simulink library "microgridLib"  (R2023a)
settings: Solver=VariableStepAuto  StartTime=0.0  StopTime=10.0  RelTol=1e-3
values from neighbouring files (symbols this model uses):
  Ts = 5.0E-5    [microgrid_system.sldd]
  Ts_Control = 5.0E-5    [microgrid_system.sldd]
undefined symbols (not defined in the file or in its folder): BR, D1, Delta, DiscIntNeverNeededParam, fnom, gcbh, I1_init, Ion, j, Lithium, Mag_V0, np, nq, Pha_V0, PQext, sps_rtmsupport, Tp1, Tp2, Tq1, Tq2, Vbase, Vmin, Vnom
libraries: slpidlib x11, spsThreePhaseSeriesRLCBranchLib x10, spsGroundLib x9, spsVoltageMeasurementLib x7, spsSeriesRLCBranchLib x7, spsControlledCurrentSourceLib x6, spsabctodq0Lib x6, spsFourierLib x5, spsPower3phInstantaneousLib x5, spsThreePhaseSeriesRLCLoadLib x4, spsThreePhaseTransformerTwoWindingsLib x4, spsThreePhaseVIMeasurementLib x3
(part 2 of 4)

== system microgridLib/Transformer ==
  Ground : spsGroundLib/Ground  LConnTagsString=a
  Shunt (Numerical Stability) : spsThreePhaseSeriesRLCBranchLib/Three-Phase Series RLC Branch  LConnTagsString=A|B|C  RConnTagsString=A|B|C  BranchType=R  Resistance=1e7  Inductance=1e-3  Capacitance=1e-6  Measurements=None
  Three-Phase Transformer (Two Windings) : spsThreePhaseTransformerTwoWindingsLib/Three-Phase Transformer (Two Windings)  Winding1Connection=Delta (D1)  Winding2Connection=Yg  CoreType=Three single-phase transformers  SetSaturation=off  Hysteresis=off  DataFile='hysteresis'  SetInitialFlux=off  Measurements=None  UNITS=pu  NominalPower=[S Freq]  Winding1=[Vp 0 0]  Winding2=[Vs Z/Ratio Z/(2*pi*Freq)]  Rm=500  Lm=500  L0=0.5  Saturation=[ 0,0 ; 0.0024,1.2 ; 1.0,1.52 ]  InitialFluxes=[ 0.8 , -0.8 , 0.7 ]  BreakLoop=off  DiscreteSolver=Trapezoidal iterative  DataType=off  TransfoNumber=1
  A : PMIOPort  Tag=PMCPort  Side=Left
  B : PMIOPort  Tag=PMCPort  Port=2  Side=Left
  C : PMIOPort  Tag=PMCPort  Port=3  Side=Left
  a : PMIOPort  Tag=PMCPort  Port=4  Side=Right
  b : PMIOPort  Tag=PMCPort  Port=5  Side=Right
  c : PMIOPort  Tag=PMCPort  Port=6  Side=Right
  connections:
  Shunt (Numerical Stability)/RConn3 -- Ground/LConn1 -- Shunt (Numerical Stability)/RConn2 -- Shunt (Numerical Stability)/RConn1
  C/RConn1 -- Shunt (Numerical Stability)/LConn3 -- Three-Phase Transformer (Two Windings)/LConn3
  Three-Phase Transformer (Two Windings)/LConn2 -- Shunt (Numerical Stability)/LConn2 -- B/RConn1
  Three-Phase Transformer (Two Windings)/LConn1 -- Shunt (Numerical Stability)/LConn1 -- A/RConn1
  c/RConn1 -- Three-Phase Transformer (Two Windings)/RConn3
  b/RConn1 -- Three-Phase Transformer (Two Windings)/RConn2
  a/RConn1 -- Three-Phase Transformer (Two Windings)/RConn1

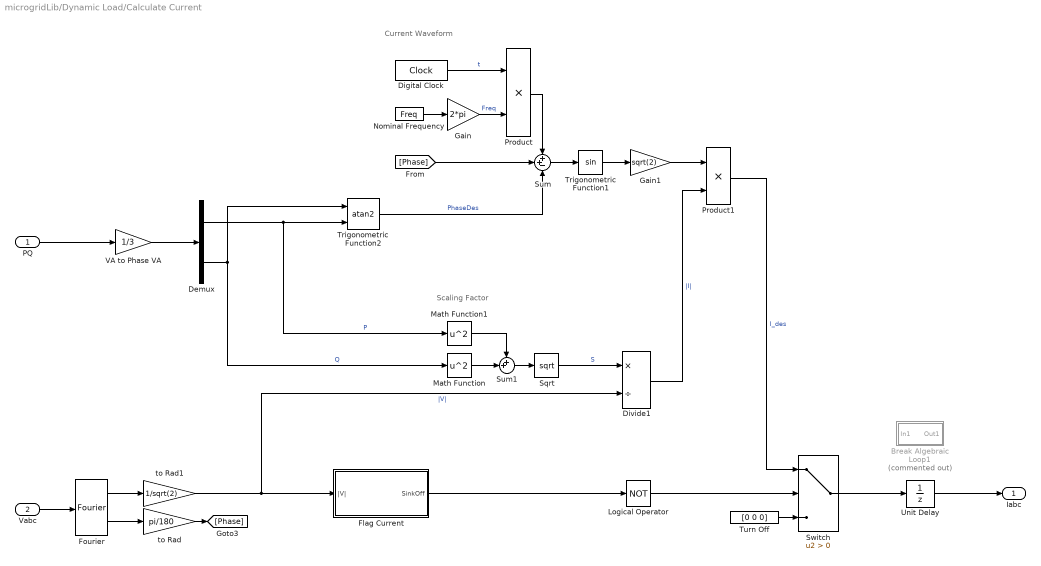
== system microgridLib/Dynamic Load/Calculate Current ==
  note: Current Waveform
  note: Scaling Factor
  PQ : Inport
  Vabc : Inport  Port=2
  Break Algebraic Loop1 : Subsystem  Commented=on  mask{Tau=Tau, Ts=Ts}
      mask prompts: Tau "Time Constant"; Ts "Sample Time"
  Demux : Demux  Outputs=2
  Digital Clock : DigitalClock  SampleTime=Ts
  Divide1 : Product  Inputs=*/
  Flag Current : Subsystem
  Fourier : spsFourierLib/Fourier  Freq=60  n=1  InInit=[Vrms*sqrt(2)/sqrt(3), 0]  Ts=Ts
  Gain : Gain  Gain=2*pi
  Gain1 : Gain  Gain=sqrt(2)
  Logical Operator : Logic  Operator=NOT  AllPortsSameDT=off  OutDataTypeStr=boolean
  Math Function : Math  Operator=square  SignedPower=on
  Math Function1 : Math  Operator=square  SignedPower=on
  Nominal Frequency : Constant  Value=Freq
  Product : Product
  Product1 : Product
  Sqrt : Sqrt
  Sum : Sum  Inputs=++-
  Sum1 : Sum  Inputs=++|
  Switch : Switch  Criteria=u2 > Threshold  SaturateOnIntegerOverflow=off  InputSameDT=off
  Trigonometric Function1 : Trigonometry
  Trigonometric Function2 : Trigonometry  Operator=atan2
  Turn Off : Constant  Value=[0 0 0]
  Unit Delay : UnitDelay  SampleTime=-1  HasFrameUpgradeWarning=on
  VA to Phase VA : Gain  Gain=1/3
  to Rad : Gain  Gain=pi/180
  to Rad1 : Gain  Gain=1/sqrt(2)
  Iabc : Outport
  wires:
  Flag Current/1(SinkOff) -> Logical Operator/1
  Unit Delay/1 -> Iabc/1
  Switch/1 -> Unit Delay/1
  Turn Off/1 -> Switch/3
  Vabc/1 -> Fourier/1
  Fourier/1 -> to Rad1/1
  Fourier/2 -> to Rad/1
  to Rad/1 -> [Phase]
  Product1/1 -> Switch/1  "I_des"
  Divide1/1 -> Product1/2  "|I|"
  Gain1/1 -> Product1/1
  to Rad1/1 -> Flag Current/1(|V|), Divide1/2  "|V|"
  Trigonometric Function1/1 -> Gain1/1
  Sum/1 -> Trigonometric Function1/1
  Math Function/1 -> Sum1/2
  Sum1/1 -> Sqrt/1
  [Phase] -> Sum/2
  Gain/1 -> Product/2  "Freq"
  Nominal Frequency/1 -> Gain/1
  Demux/2 -> Trigonometric Function2/1, Math Function/1  "Q"
  Product/1 -> Sum/1
  Math Function1/1 -> Sum1/1
  Trigonometric Function2/1 -> Sum/3  "PhaseDes"
  Digital Clock/1 -> Product/1  "t"
  Sqrt/1 -> Divide1/1  "S"
  VA to Phase VA/1 -> Demux/1
  PQ/1 -> VA to Phase VA/1
  Demux/1 -> Math Function1/1, Trigonometric Function2/2  "P"
  Logical Operator/1 -> Switch/2

== system microgridLib/Dynamic Load (Modified SPS)/Three-Phase Dynamic Load ==
  PQ : Inport
  3-PhaseDynamicLoad : PMComponent  PhysicalDomain=powersysdomain  LeftPortType=p1  RightPortType=p1  LConnTagsString=A|B  RConnTagsString=C  mask(InnerPowersysBlock){}
  Measurement list : Subsystem
  Model : spsDynamicLoadModel/Continuous  SystemSampleTime=-1  VariantActivationTime=update diagram  Latency=0  AutoFrameSizeCalculation=off
  A : PMIOPort  Side=Left
  B : PMIOPort  Port=2  Side=Left
  C : PMIOPort  Port=3  Side=Left
  m : Outport  InitialOutput=[0,0,0]
  tag scope: LibraryTag=global
  wires:
  PQ/1 -> Model/2
  Model/2 -> Measurement list/1(In1)
  [LibraryTag] -> Model/1
  Model/1 -> [LibraryTag]
  Measurement list/1(Out1) -> m/1
  connections:
  C/RConn1 -- 3-PhaseDynamicLoad/RConn1
  B/RConn1 -- 3-PhaseDynamicLoad/LConn2
  A/RConn1 -- 3-PhaseDynamicLoad/LConn1

== system microgridLib/Dynamic Load (Modified SPS)/Three-Phase Dynamic Load (custom) ==
  PQ : Inport
  3-PhaseDynamicLoad : PMComponent  PhysicalDomain=powersysdomain  LeftPortType=p1  RightPortType=p1  LConnTagsString=A|B  RConnTagsString=C  mask(InnerPowersysBlock){}
  Measurement list : Subsystem
  Model : Subsystem
  A : PMIOPort  Side=Left
  B : PMIOPort  Port=2  Side=Left
  C : PMIOPort  Port=3  Side=Left
  m : Outport  InitialOutput=[0,0,0]
  tag scope: T57_5334_5331768972450=global
  wires:
  Measurement list/1(Out1) -> m/1
  Model/1(i) -> [T57_5334_5331768972450]
  [T57_5329_5275792778477] -> Model/1(v)
  Model/2(m) -> Measurement list/1(In1)
  PQ/1 -> Model/2(PQ)
  connections:
  A/RConn1 -- 3-PhaseDynamicLoad/LConn1
  B/RConn1 -- 3-PhaseDynamicLoad/LConn2
  C/RConn1 -- 3-PhaseDynamicLoad/RConn1

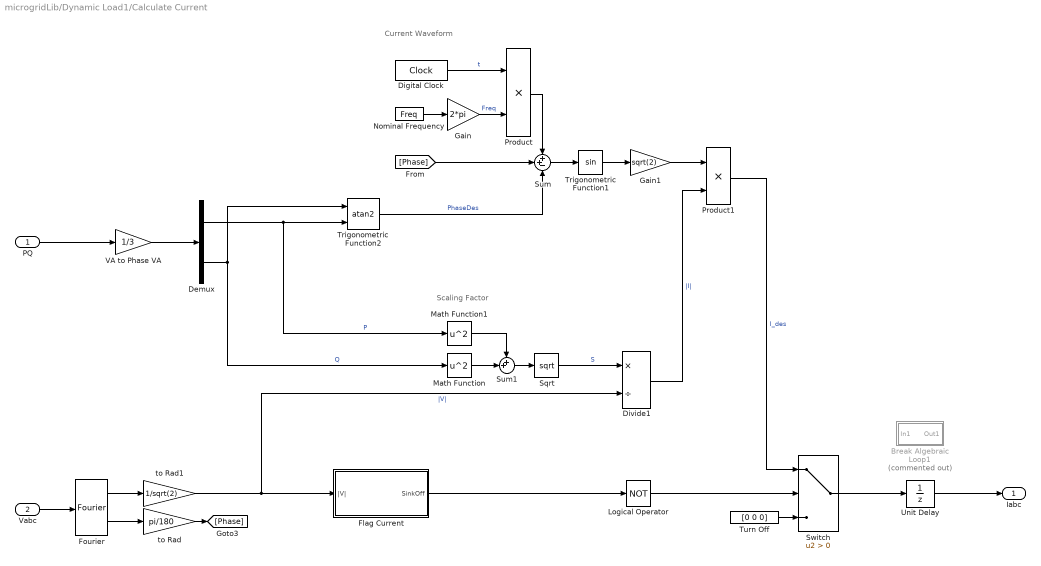
== system microgridLib/Dynamic Load1/Calculate Current ==
  note: Scaling Factor
  note: Current Waveform
  PQ : Inport
  Vabc : Inport  Port=2
  Break Algebraic Loop1 : Subsystem  Commented=on  mask{Tau=Tau, Ts=Ts}
      mask prompts: Tau "Time Constant"; Ts "Sample Time"
  Demux : Demux  Outputs=2
  Digital Clock : DigitalClock  SampleTime=Ts
  Divide1 : Product  Inputs=*/
  Flag Current : Subsystem
  Fourier : spsFourierLib/Fourier  Freq=60  n=1  InInit=[Vrms*sqrt(2)/sqrt(3), 0]  Ts=Ts
  Gain : Gain  Gain=2*pi
  Gain1 : Gain  Gain=sqrt(2)
  Logical Operator : Logic  Operator=NOT  AllPortsSameDT=off  OutDataTypeStr=boolean
  Math Function : Math  Operator=square  SignedPower=on
  Math Function1 : Math  Operator=square  SignedPower=on
  Nominal Frequency : Constant  Value=Freq
  Product : Product
  Product1 : Product
  Sqrt : Sqrt
  Sum : Sum  Inputs=++-
  Sum1 : Sum  Inputs=++|
  Switch : Switch  Criteria=u2 > Threshold  SaturateOnIntegerOverflow=off  InputSameDT=off
  Trigonometric Function1 : Trigonometry
  Trigonometric Function2 : Trigonometry  Operator=atan2
  Turn Off : Constant  Value=[0 0 0]
  Unit Delay : UnitDelay  SampleTime=-1  HasFrameUpgradeWarning=on
  VA to Phase VA : Gain  Gain=1/3
  to Rad : Gain  Gain=pi/180
  to Rad1 : Gain  Gain=1/sqrt(2)
  Iabc : Outport
  wires:
  Logical Operator/1 -> Switch/2
  Demux/1 -> Trigonometric Function2/2, Math Function1/1  "P"
  PQ/1 -> VA to Phase VA/1
  VA to Phase VA/1 -> Demux/1
  Sqrt/1 -> Divide1/1  "S"
  Digital Clock/1 -> Product/1  "t"
  Trigonometric Function2/1 -> Sum/3  "PhaseDes"
  Math Function1/1 -> Sum1/1
  Product/1 -> Sum/1
  Demux/2 -> Math Function/1, Trigonometric Function2/1  "Q"
  Nominal Frequency/1 -> Gain/1
  Gain/1 -> Product/2  "Freq"
  [Phase] -> Sum/2
  Sum1/1 -> Sqrt/1
  Math Function/1 -> Sum1/2
  Sum/1 -> Trigonometric Function1/1
  Trigonometric Function1/1 -> Gain1/1
  to Rad1/1 -> Divide1/2, Flag Current/1(|V|)  "|V|"
  Gain1/1 -> Product1/1
  Divide1/1 -> Product1/2  "|I|"
  Product1/1 -> Switch/1  "I_des"
  to Rad/1 -> [Phase]
  Fourier/2 -> to Rad/1
  Fourier/1 -> to Rad1/1
  Vabc/1 -> Fourier/1
  Turn Off/1 -> Switch/3
  Switch/1 -> Unit Delay/1
  Unit Delay/1 -> Iabc/1
  Flag Current/1(SinkOff) -> Logical Operator/1

== system microgridLib/Fault /Fault A ==
  c : Inport
  Breaker : PMComponent  PhysicalDomain=powersysdomain  LeftPortType=p1  RightPortType=p1  LConnTagsString=a  RConnTagsString=__new0  mask(InnerPowersysBlock){}
  ITAIL : Terminator
  Model : Subsystem
  Uswitch : Ground
  1 : PMIOPort  Side=Left
  2 : PMIOPort  Port=2  Side=Right
  tag scope: LibraryTag=global
  wires:
  c/1 -> Model/1("gate ")
  Uswitch/1 -> Model/2(Uswitch)
  Model/1(gate) -> [LibraryTag]
  [LibraryTag] -> ITAIL/1
  connections:
  2/RConn1 -- Breaker/RConn1
  1/RConn1 -- Breaker/LConn1

== system microgridLib/Fault /Fault B ==
  c : Inport
  Breaker : PMComponent  PhysicalDomain=powersysdomain  LeftPortType=p1  RightPortType=p1  LConnTagsString=a  RConnTagsString=__new0  mask(InnerPowersysBlock){}
  ITAIL : Terminator
  Model : Subsystem
  Uswitch : Ground
  1 : PMIOPort  Side=Left
  2 : PMIOPort  Port=2  Side=Right
  tag scope: LibraryTag=global
  wires:
  c/1 -> Model/1("gate ")
  Uswitch/1 -> Model/2(Uswitch)
  Model/1(gate) -> [LibraryTag]
  [LibraryTag] -> ITAIL/1
  connections:
  2/RConn1 -- Breaker/RConn1
  1/RConn1 -- Breaker/LConn1

== system microgridLib/Fault /Fault C ==
  c : Inport
  Breaker : PMComponent  PhysicalDomain=powersysdomain  LeftPortType=p1  RightPortType=p1  LConnTagsString=a  RConnTagsString=__new0  mask(InnerPowersysBlock){}
  ITAIL : Terminator
  Model : Subsystem
  Uswitch : Ground
  1 : PMIOPort  Side=Left
  2 : PMIOPort  Port=2  Side=Right
  tag scope: LibraryTag=global
  wires:
  c/1 -> Model/1("gate ")
  Uswitch/1 -> Model/2(Uswitch)
  Model/1(gate) -> [LibraryTag]
  [LibraryTag] -> ITAIL/1
  connections:
  2/RConn1 -- Breaker/RConn1
  1/RConn1 -- Breaker/LConn1

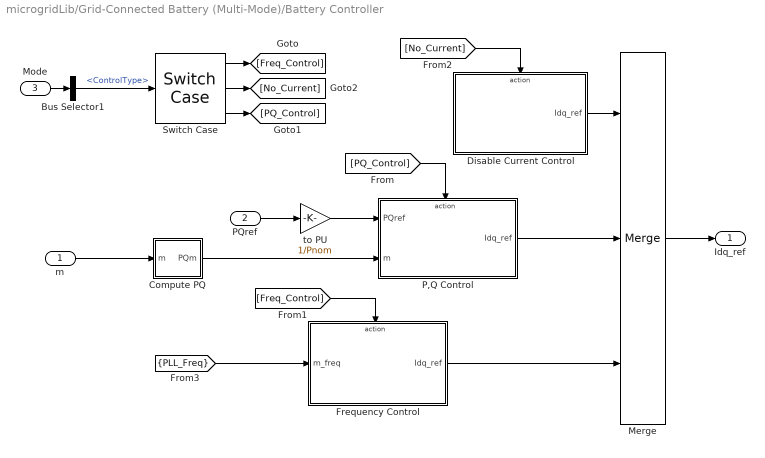
== system microgridLib/Grid-Connected Battery (Multi-Mode)/Battery Controller ==
  m : Inport
  PQref : Inport  Port=2
  Mode : Inport  Port=3  SampleTime=Ts_Control
  Bus Selector1 : BusSelector  OutputSignals=ControlType
  Compute PQ : Subsystem
  Disable Current Control : Subsystem  TreatAsAtomicUnit=on
  "Frequency Control " : Subsystem  TreatAsAtomicUnit=on
  Merge : Merge  Inputs=3
  "P,Q Control " : Subsystem  TreatAsAtomicUnit=on
  Switch Case : SwitchCase  CaseConditions={1,2}
  to PU : Gain  Gain=1/Pnom
  Idq_ref : Outport
  wires:
  [PLL_Freq] -> "Frequency Control "/1(m_freq)
  Disable Current Control/1(Idq_ref) -> Merge/1
  "P,Q Control "/1(Idq_ref) -> Merge/2
  [No_Current] -> Disable Current Control/Action
  Switch Case/2 -> [No_Current]
  Bus Selector1/1 -> Switch Case/1  "<ControlType>"
  Mode/1 -> Bus Selector1/1
  "Frequency Control "/1(Idq_ref) -> Merge/3
  to PU/1 -> "P,Q Control "/1(PQref)
  Switch Case/1 -> [Freq_Control]
  Switch Case/3 -> [PQ_Control]
  [PQ_Control] -> "P,Q Control "/Action
  m/1 -> Compute PQ/1(m)
  [Freq_Control] -> "Frequency Control "/Action
  PQref/1 -> to PU/1
  Compute PQ/1(PQm) -> "P,Q Control "/2(m)
  Merge/1 -> Idq_ref/1

== system microgridLib/Grid-Connected Battery (Multi-Mode)/DC Link ==
  C1 : spsSeriesRLCBranchLib/Series RLC Branch  LConnTagsString=__new0  RConnTagsString=__new0  BranchType=C  Resistance=1.0  Inductance=1.0  SetiL0=off  InitialCurrent=0  Capacitance=Clink  Setx0=on  InitialVoltage=Vnom_dc/2  Measurements=None
  C2 : spsSeriesRLCBranchLib/Series RLC Branch  LConnTagsString=__new0  RConnTagsString=__new0  BranchType=C  Resistance=1e5  Inductance=1.0  SetiL0=off  InitialCurrent=0  Capacitance=Clink  Setx0=on  InitialVoltage=Vnom_dc/2  Measurements=None
  PV+ : PMIOPort  Side=Left
  PV-- : PMIOPort  Port=2  Side=Left
  Inv+ : PMIOPort  Port=3  Side=Right
  N : PMIOPort  Port=4  Side=Right
  Inv-- : PMIOPort  Port=5  Side=Right
  connections:
  Inv--/RConn1 -- PV--/RConn1 -- C2/RConn1
  C1/RConn1 -- N/RConn1 -- C2/LConn1
  Inv+/RConn1 -- PV+/RConn1 -- C1/LConn1

== system microgridLib/Grid-Connected Battery (Multi-Mode)/Grid Inverter ==
  note: Harmonic Filter
  Uref : Inport
  10 kvar : spsThreePhaseSeriesRLCLoadLib/Three-Phase Series RLC Load  LConnTagsString=A|B|C  Configuration=Delta  NominalVoltage=Vnom_sec  Vabc=[1e3 1e3 1e3]  Vabcp=[1e3 1e3 1e3]  NominalFrequency=Fnom  UnbalancedPower=off  ActivePower=Pc  InductivePower=0  CapacitivePower=Qc  Pabc=[10e3 9e3 11e3]  QLabc=[100 90 110]  QCabc=[100 90 110]  Pabcp=[10e3 9e3 11e3]  QLabcp=[100 90 110]  QCabcp=[100 90 110]  Measurements=None  LoadType=constant Z
  100 kVA 260V / 25 kV : spsThreePhaseTransformerTwoWindingsLib/Three-Phase Transformer (Two Windings)  Winding1Connection=Yg  Winding2Connection=Delta (D1)  CoreType=Three single-phase transformers  SetSaturation=off  Hysteresis=off  DataFile='hysteresis'  SetInitialFlux=off  Measurements=None  UNITS=pu  NominalPower=[Pnom Fnom ]  Winding1=[ Vnom_prim , Rxf/2 , Lxf/2 ]  Winding2=[ Vnom_sec , Rxf/2 , Lxf/2 ]  Rm=200  Lm=200  L0=0.5  Saturation=[ 0,0 ; 0.0024,1.2 ; 1.0,1.52 ]  InitialFluxes=[ 0.8 , -0.8 , 0.7 ]  BreakLoop=off  DiscreteSolver=Trapezoidal iterative  DataType=off  TransfoNumber=0
  B1 : spsThreePhaseVIMeasurementLib/Three-Phase V-I Measurement  VoltageMeasurement=phase-to-ground  SetLabelV=off  LabelV=Vabc_B1  Vpu=off  VpuLL=off  CurrentMeasurement=yes  SetLabelI=off  LabelI=Iabc_B1  Ipu=off  Pbase=100e6  Vbase=500e3  OutputType=Magnitude  PhasorSimulation=off  PSBequivalent=0
  Bus Creator : BusCreator  Inputs=2
  Ground : Ground
  L : spsThreePhaseSeriesRLCBranchLib/Three-Phase Series RLC Branch  LConnTagsString=A|B|C  RConnTagsString=A|B|C  BranchType=RL  Resistance=Rchoke*Zbase  Inductance=Lchoke*Zbase/(2*pi*Fnom)  Capacitance=inf  Measurements=None
  Three-Level NPC Converter : spsThreeLevelNPCConverterLib/Three-Level NPC Converter  ModelType=Average model (Uref-controlled)  Ron=1e-3  Rs=1e6  Cs=inf  Vforward=[0,0]  Ron_Diode=1e-3  Rs_Diode=1e6  Cs_Diode=inf  Vf_Diode=1e-3  Rs_CurrentSource=inf  Ron_ACsource=1e-3
      settings: LibrarySourceBlock=|
      | sps_lib/Power Electronics/Three-Level
      | NPC Converter
  Inv+ : PMIOPort  Side=Left
  N : PMIOPort  Port=2  Side=Left
  Inv-- : PMIOPort  Port=3  Side=Left
  A : PMIOPort  Port=4  Side=Right
  B : PMIOPort  Port=5  Side=Right
  C : PMIOPort  Port=6  Side=Right
  m : Outport
  wires:
  Uref/1 -> Three-Level NPC Converter/1
  B1/1 -> Bus Creator/1  "Vabc"
  B1/2 -> Bus Creator/2  "Iabc"
  Bus Creator/1 -> m/1
  Ground/1 -> Three-Level NPC Converter/2
  connections:
  B1/RConn3 -- C/RConn1
  B1/RConn2 -- B/RConn1
  B1/RConn1 -- A/RConn1
  10 kvar/LConn1 -- 100 kVA 260V / 25 kV/RConn1 -- L/RConn1
  Three-Level NPC Converter/RConn1 -- Inv+/RConn1
  Three-Level NPC Converter/RConn3 -- Inv--/RConn1
  L/RConn3 -- 100 kVA 260V / 25 kV/RConn3 -- 10 kvar/LConn3
  L/RConn2 -- 100 kVA 260V / 25 kV/RConn2 -- 10 kvar/LConn2
  100 kVA 260V / 25 kV/LConn3 -- B1/LConn3
  100 kVA 260V / 25 kV/LConn2 -- B1/LConn2
  100 kVA 260V / 25 kV/LConn1 -- B1/LConn1
  Three-Level NPC Converter/LConn1 -- L/LConn1
  Three-Level NPC Converter/LConn2 -- L/LConn2
  Three-Level NPC Converter/LConn3 -- L/LConn3
  N/RConn1 -- Three-Level NPC Converter/RConn2

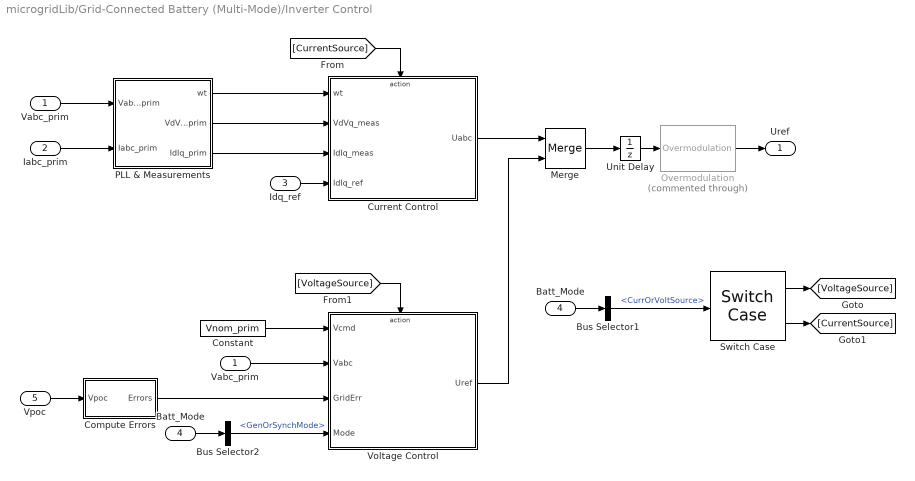
== system microgridLib/Grid-Connected Battery (Multi-Mode)/Inverter Control ==
  Vabc_prim : Inport  PortDimensions=3
  Iabc_prim : Inport  Port=2  PortDimensions=3
  Idq_ref : Inport  Port=3
  Batt_Mode : Inport  Port=4  PortDimensions=1  SampleTime=Ts_Control
  Vpoc : Inport  Port=5
  "Batt_Mode " : InportShadow  Port=4  PortDimensions=1  SampleTime=Ts_Control
  Bus Selector1 : BusSelector  OutputSignals=Bus_Batt_Mode.CurrOrVoltSource
  Bus Selector2 : BusSelector  OutputSignals=Bus_Batt_Mode.GenOrSynchMode
  Compute Errors : Subsystem
  Constant : Constant  Value=Vnom_prim
  Current Control : Subsystem  TreatAsAtomicUnit=on
  Merge : Merge
  Overmodulation : spsOvermodulationLib/Overmodulation  Commented=through  OverModType=Flat top
      settings: LibrarySourceBlock=sps_lib/Power Electronics/Power Electronics Control/Overmodulation
  PLL & Measurements : Subsystem
  Switch Case : SwitchCase
  Unit Delay : UnitDelay  SampleTime=Ts_Control  HasFrameUpgradeWarning=on
  "Vabc_prim " : InportShadow  PortDimensions=3
  Voltage Control : Subsystem  TreatAsAtomicUnit=on
  Uref : Outport
  wires:
  "Batt_Mode "/1 -> Bus Selector2/1
  Bus Selector2/1 -> Voltage Control/4(Mode)  "<GenOrSynchMode>"
  Bus Selector1/1 -> Switch Case/1  "<CurrOrVoltSource>"
  Compute Errors/1(Errors) -> Voltage Control/3(GridErr)
  Vpoc/1 -> Compute Errors/1(Vpoc)
  Batt_Mode/1 -> Bus Selector1/1
  Unit Delay/1 -> Overmodulation/1
  Overmodulation/1 -> Uref/1
  "Vabc_prim "/1 -> Voltage Control/2(Vabc)
  Constant/1 -> Voltage Control/1(Vcmd)
  Merge/1 -> Unit Delay/1
  Voltage Control/1(Uref) -> Merge/2
  Current Control/1(Uabc) -> Merge/1
  Idq_ref/1 -> Current Control/4(IdIq_ref)
  PLL & Measurements/1(wt) -> Current Control/1(wt)
  PLL & Measurements/2(VdVq_prim) -> Current Control/2(VdVq_meas)
  PLL & Measurements/3(IdIq_prim) -> Current Control/3(IdIq_meas)
  Iabc_prim/1 -> PLL & Measurements/2(Iabc_prim)
  Vabc_prim/1 -> PLL & Measurements/1(Vabc_prim)
  [VoltageSource] -> Voltage Control/Action
  [CurrentSource] -> Current Control/Action
  Switch Case/1 -> [VoltageSource]
  Switch Case/2 -> [CurrentSource]

== system microgridLib/Grid-Connected Battery (Multi-Mode)/Measures ==
  Grid : Inport
  Battery : Inport  Port=2
  Bus Creator : BusCreator  Inputs=2
  Bus Creator1 : BusCreator  Inputs=4
  Bus Selector2 : BusSelector  OutputSignals=Vabc,Iabc
  "Power (3ph, Instantaneous)" : spsPower3phInstantaneousLib/Power (3ph, Instantaneous)
  m : Outport
  wires:
  Bus Creator1/1 -> Bus Creator/1  "Grid"
  "Power (3ph, Instantaneous)"/2 -> Bus Creator1/4  "Q"
  Grid/1 -> Bus Selector2/1
  Battery/1 -> Bus Creator/2  "Battery"
  Bus Creator/1 -> m/1
  "Power (3ph, Instantaneous)"/1 -> Bus Creator1/3  "P"
  Bus Selector2/2 -> Bus Creator1/2, "Power (3ph, Instantaneous)"/2  "<Iabc>"
  Bus Selector2/1 -> Bus Creator1/1, "Power (3ph, Instantaneous)"/1  "<Vabc>"

== system microgridLib/Grid-Connected Battery (Simple PQ Only)/Battery Controller ==
  m : Inport
  PQref : Inport  Port=2
  Compute PQ : Subsystem
  "P,Q Control " : Subsystem  TreatAsAtomicUnit=on
  to PU : Gain  Gain=1/Pnom
  Idq_ref : Outport
  wires:
  "P,Q Control "/1(Idq_ref) -> Idq_ref/1
  to PU/1 -> "P,Q Control "/1(PQref)
  m/1 -> Compute PQ/1(m)
  PQref/1 -> to PU/1
  Compute PQ/1(PQm) -> "P,Q Control "/2(m)

== system microgridLib/Grid-Connected Battery (Simple PQ Only)/DC Link ==
  C1 : spsSeriesRLCBranchLib/Series RLC Branch  LConnTagsString=__new0  RConnTagsString=__new0  BranchType=C  Resistance=1.0  Inductance=1.0  SetiL0=off  InitialCurrent=0  Capacitance=Clink  Setx0=on  InitialVoltage=Vnom_dc/2  Measurements=None
  C2 : spsSeriesRLCBranchLib/Series RLC Branch  LConnTagsString=__new0  RConnTagsString=__new0  BranchType=C  Resistance=1e5  Inductance=1.0  SetiL0=off  InitialCurrent=0  Capacitance=Clink  Setx0=on  InitialVoltage=Vnom_dc/2  Measurements=None
  PV+ : PMIOPort  Side=Left
  PV-- : PMIOPort  Port=2  Side=Left
  Inv+ : PMIOPort  Port=3  Side=Right
  N : PMIOPort  Port=4  Side=Right
  Inv-- : PMIOPort  Port=5  Side=Right
  connections:
  Inv--/RConn1 -- PV--/RConn1 -- C2/RConn1
  C1/RConn1 -- N/RConn1 -- C2/LConn1
  Inv+/RConn1 -- PV+/RConn1 -- C1/LConn1

== system microgridLib/Grid-Connected Battery (Simple PQ Only)/Grid Inverter ==
  note: Harmonic Filter
  Uref : Inport
  10 kvar : spsThreePhaseSeriesRLCLoadLib/Three-Phase Series RLC Load  LConnTagsString=A|B|C  Configuration=Delta  NominalVoltage=Vnom_sec  Vabc=[1e3 1e3 1e3]  Vabcp=[1e3 1e3 1e3]  NominalFrequency=Fnom  UnbalancedPower=off  ActivePower=Pc  InductivePower=0  CapacitivePower=Qc  Pabc=[10e3 9e3 11e3]  QLabc=[100 90 110]  QCabc=[100 90 110]  Pabcp=[10e3 9e3 11e3]  QLabcp=[100 90 110]  QCabcp=[100 90 110]  Measurements=None  LoadType=constant Z
  100 kVA 260V / 25 kV : spsThreePhaseTransformerTwoWindingsLib/Three-Phase Transformer (Two Windings)  Winding1Connection=Yg  Winding2Connection=Delta (D1)  CoreType=Three single-phase transformers  SetSaturation=off  Hysteresis=off  DataFile='hysteresis'  SetInitialFlux=off  Measurements=None  UNITS=pu  NominalPower=[Pnom Fnom ]  Winding1=[ Vnom_prim , Rxf/2 , Lxf/2 ]  Winding2=[ Vnom_sec , Rxf/2 , Lxf/2 ]  Rm=200  Lm=200  L0=0.5  Saturation=[ 0,0 ; 0.0024,1.2 ; 1.0,1.52 ]  InitialFluxes=[ 0.8 , -0.8 , 0.7 ]  BreakLoop=off  DiscreteSolver=Trapezoidal iterative  DataType=off  TransfoNumber=0
  B1 : spsThreePhaseVIMeasurementLib/Three-Phase V-I Measurement  VoltageMeasurement=phase-to-ground  SetLabelV=off  LabelV=Vabc_B1  Vpu=off  VpuLL=off  CurrentMeasurement=yes  SetLabelI=off  LabelI=Iabc_B1  Ipu=off  Pbase=100e6  Vbase=500e3  OutputType=Magnitude  PhasorSimulation=off  PSBequivalent=0
  Bus Creator : BusCreator  Inputs=2
  Ground : Ground
  L : spsThreePhaseSeriesRLCBranchLib/Three-Phase Series RLC Branch  LConnTagsString=A|B|C  RConnTagsString=A|B|C  BranchType=RL  Resistance=Rchoke*Zbase  Inductance=Lchoke*Zbase/(2*pi*Fnom)  Capacitance=inf  Measurements=None
  Three-Level NPC Converter : spsThreeLevelNPCConverterLib/Three-Level NPC Converter  ModelType=Average model (Uref-controlled)  Ron=1e-3  Rs=1e6  Cs=inf  Vforward=[0,0]  Ron_Diode=1e-3  Rs_Diode=1e6  Cs_Diode=inf  Vf_Diode=1e-3  Rs_CurrentSource=inf  Ron_ACsource=1e-3
      settings: LibrarySourceBlock=|
      | sps_lib/Power Electronics/Three-Level
      | NPC Converter
  Inv+ : PMIOPort  Side=Left
  N : PMIOPort  Port=2  Side=Left
  Inv-- : PMIOPort  Port=3  Side=Left
  A : PMIOPort  Port=4  Side=Right
  B : PMIOPort  Port=5  Side=Right
  C : PMIOPort  Port=6  Side=Right
  m : Outport
  wires:
  Uref/1 -> Three-Level NPC Converter/1
  B1/1 -> Bus Creator/1  "Vabc"
  B1/2 -> Bus Creator/2  "Iabc"
  Bus Creator/1 -> m/1
  Ground/1 -> Three-Level NPC Converter/2
  connections:
  B1/RConn3 -- C/RConn1
  B1/RConn2 -- B/RConn1
  B1/RConn1 -- A/RConn1
  10 kvar/LConn1 -- 100 kVA 260V / 25 kV/RConn1 -- L/RConn1
  Three-Level NPC Converter/RConn1 -- Inv+/RConn1
  Three-Level NPC Converter/RConn3 -- Inv--/RConn1
  L/RConn3 -- 100 kVA 260V / 25 kV/RConn3 -- 10 kvar/LConn3
  L/RConn2 -- 100 kVA 260V / 25 kV/RConn2 -- 10 kvar/LConn2
  100 kVA 260V / 25 kV/LConn3 -- B1/LConn3
  100 kVA 260V / 25 kV/LConn2 -- B1/LConn2
  100 kVA 260V / 25 kV/LConn1 -- B1/LConn1
  Three-Level NPC Converter/LConn1 -- L/LConn1
  Three-Level NPC Converter/LConn2 -- L/LConn2
  Three-Level NPC Converter/LConn3 -- L/LConn3
  N/RConn1 -- Three-Level NPC Converter/RConn2

== system microgridLib/Grid-Connected Battery (Simple PQ Only)/Inverter Control ==
  Vabc_prim : Inport  PortDimensions=3
  Iabc_prim : Inport  Port=2  PortDimensions=3
  Idq_ref : Inport  Port=3
  Current Control : Subsystem  TreatAsAtomicUnit=on
  Overmodulation : spsOvermodulationLib/Overmodulation  OverModType=Flat top
      settings: LibrarySourceBlock=sps_lib/Power Electronics/Power Electronics Control/Overmodulation
  PLL & Measurements : Subsystem
  Unit Delay : UnitDelay  SampleTime=Ts_Control  HasFrameUpgradeWarning=on
  Uref : Outport
  wires:
  Unit Delay/1 -> Overmodulation/1
  Overmodulation/1 -> Uref/1
  Current Control/1(Uabc) -> Unit Delay/1
  Idq_ref/1 -> Current Control/4(IdIq_ref)
  PLL & Measurements/1(wt) -> Current Control/1(wt)
  PLL & Measurements/2(VdVq_prim) -> Current Control/2(VdVq_meas)
  PLL & Measurements/3(IdIq_prim) -> Current Control/3(IdIq_meas)
  Iabc_prim/1 -> PLL & Measurements/2(Iabc_prim)
  Vabc_prim/1 -> PLL & Measurements/1(Vabc_prim)

== system microgridLib/Grid-Connected Battery (Simple PQ Only)/Measures ==
  Grid : Inport
  Battery : Inport  Port=2
  Bus Creator : BusCreator  Inputs=2
  Bus Creator1 : BusCreator  Inputs=4
  Bus Selector2 : BusSelector  OutputSignals=Vabc,Iabc
  "Power (3ph, Instantaneous)" : spsPower3phInstantaneousLib/Power (3ph, Instantaneous)
  m : Outport
  wires:
  Bus Creator1/1 -> Bus Creator/1  "Grid"
  "Power (3ph, Instantaneous)"/2 -> Bus Creator1/4  "Q"
  Grid/1 -> Bus Selector2/1
  Battery/1 -> Bus Creator/2  "Battery"
  Bus Creator/1 -> m/1
  "Power (3ph, Instantaneous)"/1 -> Bus Creator1/3  "P"
  Bus Selector2/2 -> Bus Creator1/2, "Power (3ph, Instantaneous)"/2  "<Iabc>"
  Bus Selector2/1 -> Bus Creator1/1, "Power (3ph, Instantaneous)"/1  "<Vabc>"

== system microgridLib/Grid-Connected PV Array/DC Link ==
  C1 : spsSeriesRLCBranchLib/Series RLC Branch  LConnTagsString=__new0  RConnTagsString=__new0  BranchType=C  Resistance=1.0  Inductance=1.0  SetiL0=off  InitialCurrent=0  Capacitance=Clink  Setx0=on  InitialVoltage=Vnom_dc/2  Measurements=None
  C2 : spsSeriesRLCBranchLib/Series RLC Branch  LConnTagsString=__new0  RConnTagsString=__new0  BranchType=C  Resistance=1e5  Inductance=1.0  SetiL0=off  InitialCurrent=0  Capacitance=Clink  Setx0=on  InitialVoltage=Vnom_dc/2  Measurements=None
  "Vdc " : spsVoltageMeasurementLib/Voltage Measurement  Tag=PoWeRsYsTeMmEaSuReMeNt  PhasorSimulation=off  OutputType=Magnitude  PSBequivalent=0
  PV+ : PMIOPort  Side=Left
  PV-- : PMIOPort  Port=2  Side=Left
  Inv+ : PMIOPort  Port=3  Side=Right
  N : PMIOPort  Port=4  Side=Right
  Inv-- : PMIOPort  Port=5  Side=Right
  Vdc : Outport
  wires:
  "Vdc "/1 -> Vdc/1
  connections:
  C1/LConn1 -- PV+/RConn1 -- "Vdc "/LConn1 -- Inv+/RConn1
  C2/LConn1 -- N/RConn1 -- C1/RConn1
  "Vdc "/LConn2 -- C2/RConn1 -- PV--/RConn1 -- Inv--/RConn1

== system microgridLib/Grid-Connected PV Array/Grid Inverter ==
  note: Harmonic Filter
  Uref : Inport
  10 kvar : spsThreePhaseSeriesRLCLoadLib/Three-Phase Series RLC Load  LConnTagsString=A|B|C  Configuration=Delta  NominalVoltage=Vnom_sec  Vabc=[1e3 1e3 1e3]  Vabcp=[1e3 1e3 1e3]  NominalFrequency=Fnom  UnbalancedPower=off  ActivePower=Pc  InductivePower=0  CapacitivePower=Qc  Pabc=[10e3 9e3 11e3]  QLabc=[100 90 110]  QCabc=[100 90 110]  Pabcp=[10e3 9e3 11e3]  QLabcp=[100 90 110]  QCabcp=[100 90 110]  Measurements=None  LoadType=constant Z
  100 kVA 260V / 25 kV : spsThreePhaseTransformerTwoWindingsLib/Three-Phase Transformer (Two Windings)  Winding1Connection=Yg  Winding2Connection=Delta (D1)  CoreType=Three single-phase transformers  SetSaturation=off  Hysteresis=off  DataFile='hysteresis'  SetInitialFlux=off  Measurements=None  UNITS=pu  NominalPower=[Pnom Fnom ]  Winding1=[ Vnom_prim , Rxf/2 , Lxf/2 ]  Winding2=[ Vnom_sec , Rxf/2 , Lxf/2 ]  Rm=200  Lm=200  L0=0.5  Saturation=[ 0,0 ; 0.0024,1.2 ; 1.0,1.52 ]  InitialFluxes=[ 0.8 , -0.8 , 0.7 ]  BreakLoop=off  DiscreteSolver=Trapezoidal iterative  DataType=off  TransfoNumber=0
  B1 : spsThreePhaseVIMeasurementLib/Three-Phase V-I Measurement  VoltageMeasurement=phase-to-ground  SetLabelV=off  LabelV=Vabc_B1  Vpu=off  VpuLL=off  CurrentMeasurement=yes  SetLabelI=off  LabelI=Iabc_B1  Ipu=off  Pbase=100e6  Vbase=500e3  OutputType=Magnitude  PhasorSimulation=off  PSBequivalent=0
  Bus Creator : BusCreator  Inputs=2
  Ground : Ground
  L : spsThreePhaseSeriesRLCBranchLib/Three-Phase Series RLC Branch  LConnTagsString=A|B|C  RConnTagsString=A|B|C  BranchType=RL  Resistance=Rchoke*Zbase  Inductance=Lchoke*Zbase/(2*pi*Fnom)  Capacitance=inf  Measurements=None
  Three-Level NPC Converter : spsThreeLevelNPCConverterLib/Three-Level NPC Converter  ModelType=Average model (Uref-controlled)  Ron=1e-3  Rs=1e6  Cs=inf  Vforward=[0,0]  Ron_Diode=1e-3  Rs_Diode=1e6  Cs_Diode=inf  Vf_Diode=1e-3  Rs_CurrentSource=inf  Ron_ACsource=1e-3
      settings: LibrarySourceBlock=|
      | sps_lib/Power Electronics/Three-Level
      | NPC Converter
  Inv+ : PMIOPort  Side=Left
  N : PMIOPort  Port=2  Side=Left
  Inv-- : PMIOPort  Port=3  Side=Left
  A : PMIOPort  Port=4  Side=Right
  B : PMIOPort  Port=5  Side=Right
  C : PMIOPort  Port=6  Side=Right
  m : Outport
  wires:
  Ground/1 -> Three-Level NPC Converter/2
  Bus Creator/1 -> m/1
  B1/2 -> Bus Creator/2  "Iabc"
  B1/1 -> Bus Creator/1  "Vabc"
  Uref/1 -> Three-Level NPC Converter/1
  connections:
  N/RConn1 -- Three-Level NPC Converter/RConn2
  Three-Level NPC Converter/LConn3 -- L/LConn3
  Three-Level NPC Converter/LConn2 -- L/LConn2
  Three-Level NPC Converter/LConn1 -- L/LConn1
  100 kVA 260V / 25 kV/LConn1 -- B1/LConn1
  100 kVA 260V / 25 kV/LConn2 -- B1/LConn2
  100 kVA 260V / 25 kV/LConn3 -- B1/LConn3
  10 kvar/LConn2 -- 100 kVA 260V / 25 kV/RConn2 -- L/RConn2
  10 kvar/LConn3 -- 100 kVA 260V / 25 kV/RConn3 -- L/RConn3
  Three-Level NPC Converter/RConn3 -- Inv--/RConn1
  Three-Level NPC Converter/RConn1 -- Inv+/RConn1
  L/RConn1 -- 100 kVA 260V / 25 kV/RConn1 -- 10 kvar/LConn1
  B1/RConn1 -- A/RConn1
  B1/RConn2 -- B/RConn1
  B1/RConn3 -- C/RConn1

== system microgridLib/Grid-Connected PV Array/Inverter Control ==
  On : Inport  PortDimensions=1
  Vabc_prim : Inport  Port=2  PortDimensions=3
  Iabc_prim : Inport  Port=3  PortDimensions=3
  V_PV : Inport  Port=4  PortDimensions=1
  I_PV : Inport  Port=5  PortDimensions=1
  Vdc_meas : Inport  Port=6  PortDimensions=1
  Current Regulator : Subsystem
  Iq_ref : Constant  Value=0
  MPPT Parameters : Subsystem
  "MPPT Controller using Perturbe & Observe technique " : MATLAB Function  TreatAsAtomicUnit=on
  Mux : Mux  Inputs=2
  Overmodulation : spsOvermodulationLib/Overmodulation  OverModType=Flat top
      settings: LibrarySourceBlock=sps_lib/Power Electronics/Power Electronics Control/Overmodulation
  PLL & Measurements : Subsystem
  Switch : Switch  Criteria=u2 ~= 0  SaturateOnIntegerOverflow=off  InputSameDT=off
  Uabc_ref Generation max (m) = 1 : Subsystem
  Unit Delay : UnitDelay  SampleTime=Ts_Control  HasFrameUpgradeWarning=on
  VDC Regulator : Subsystem
  Vnom_dc1 : Constant  Value=Vnom_dc
  Uref : Outport
  wires:
  PLL & Measurements/1(wt) -> Uabc_ref Generation max (m) = 1/1(wt)
  Current Regulator/1(VdVq_conv) -> Uabc_ref Generation max (m) = 1/2(VdVq_conv)
  Iq_ref/1 -> Mux/2
  Mux/1 -> Current Regulator/3(IdIq_ref)
  PLL & Measurements/3(IdIq_prim) -> Current Regulator/2(IdIq_meas)
  PLL & Measurements/2(VdVq_prim) -> Current Regulator/1(VdVq_meas)
  Vabc_prim/1 -> PLL & Measurements/1(Vabc_prim)
  Iabc_prim/1 -> PLL & Measurements/2(Iabc_prim)
  Overmodulation/1 -> Uref/1
  Vdc_meas/1 -> VDC Regulator/1(Vdc_meas)
  VDC Regulator/1(Id_ref) -> Mux/1
  V_PV/1 -> "MPPT Controller using Perturbe & Observe technique "/3(V)
  I_PV/1 -> "MPPT Controller using Perturbe & Observe technique "/4(I)
  MPPT Parameters/1(Param) -> "MPPT Controller using Perturbe & Observe technique "/1(Param)
  On/1 -> "MPPT Controller using Perturbe & Observe technique "/2(Enabled), Switch/2
  Unit Delay/1 -> Overmodulation/1
  "MPPT Controller using Perturbe & Observe technique "/1(D) -> Switch/1
  Switch/1 -> VDC Regulator/2(Vdc_ref)
  Vnom_dc1/1 -> Switch/3
  Uabc_ref Generation max (m) = 1/1(Uabc_ref) -> Unit Delay/1

== system microgridLib/Grid-Connected PV Array/Measures ==
  Grid : Inport
  PV : Inport  Port=2
  Bus Creator : BusCreator  Inputs=2
  Bus Creator1 : BusCreator  Inputs=4
  Bus Selector2 : BusSelector  OutputSignals=Vabc,Iabc
  "Power (3ph, Instantaneous)" : spsPower3phInstantaneousLib/Power (3ph, Instantaneous)
  m : Outport
  wires:
  Bus Selector2/1 -> "Power (3ph, Instantaneous)"/1, Bus Creator1/1  "<Vabc>"
  Bus Selector2/2 -> "Power (3ph, Instantaneous)"/2, Bus Creator1/2  "<Iabc>"
  "Power (3ph, Instantaneous)"/1 -> Bus Creator1/3  "P"
  Bus Creator/1 -> m/1
  PV/1 -> Bus Creator/2  "PV"
  Grid/1 -> Bus Selector2/1
  "Power (3ph, Instantaneous)"/2 -> Bus Creator1/4  "Q"
  Bus Creator1/1 -> Bus Creator/1  "Grid"

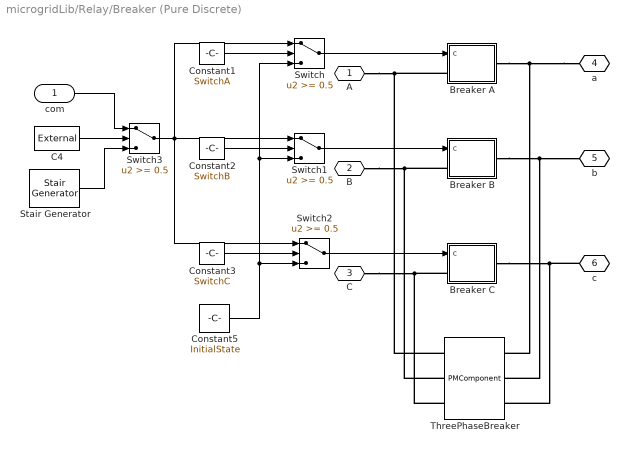
== system microgridLib/Relay/Breaker (Pure Discrete) ==
  com : Inport
  Breaker A : Subsystem  DialogController=POWERSYS.PowerSysDialog  LoadFcn=sps_rtmsupport('LoadFcn',gcbh);  StartFcn=sps_rtmsupport('StartFcn',gcbh);  StopFcn=sps_rtmsupport('StopFcn',gcbh);  mask(Breaker){InitialState=InitialState, SwitchingTimes=[ 1/60  5/60 ], External=on, BreakerResistance=BreakerResistance, SnubberResistance=SnubberResistance, SnubberCapacitance=SnubberCapacitance, Measurements=None, MoreParameters=off, NoBreakLoop=off}
      mask prompts: InitialState "Initial status:"; SwitchingTimes "Switching times (s):"; BreakerResistance "Breaker resistance Ron (Ohm):"; SnubberResistance "Snubber resistance Rs (Ohm):"; SnubberCapacitance "Snubber capacitance Cs (F):"; MoreParameters "obsolete"; NoBreakLoop "Enable zero crossing detection (create an algebraic loop)"
      mask help: Implements a circuit breaker. When the external switching time option is selected, a Simulink logical signal is used to control the breaker operation.
      mask init: same as microgridLib/Fault /Fault A
      settings: CopyFcn=sps_rtmsupport('CopyFcn',gcbh); powericon('SwitchesCopyFcn','Breaker',gcb)  DeleteFcn=sps_rtmsupport('DeleteFcn',gcbh);  UndoDeleteFcn=sps_rtmsupport('UndoDeleteFcn',gcbh);  ModelCloseFcn=sps_rtmsupport('ModelCloseFcn',gcbh);  PreSaveFcn=sps_rtmsupport('PreSaveFcn',gcbh);  PostSaveFcn=sps_rtmsupport('PostSaveFcn',gcbh);  NameChangeFcn=sps_rtmsupport('NameChangeFcn',gcbh);  PreCopyFcn=sps_rtmsupport('PreCopyFcn',gcbh);  OpenFcn=sps_rtmsupport('OpenFcn',gcbh, [3 7 8 9]);  CloseFcn=sps_rtmsupport('CloseFcn',gcbh);  PreDeleteFcn=sps_rtmsupport('PreDeleteFcn',gcbh);
      mask Help: helpview(psbhelp);
      mask Callback External: powericon('BreakerCback',gcb);
      mask Callback BreakerResistance: powericon('SwitchesEnables',gcb,'Breaker');
      mask TypeOptions Measurements: None | Branch voltage | Branch current | Branch voltage and current
      mask Display: % plot(X.p1,Y.p1,X.p2,Y.p2,X.p3,Y.p3,X.p4,Y.p4,X.p5,Y.p5,X.p6,Y.p6)
  Breaker B : Subsystem  DialogController=POWERSYS.PowerSysDialog  LoadFcn=sps_rtmsupport('LoadFcn',gcbh);  StartFcn=sps_rtmsupport('StartFcn',gcbh);  StopFcn=sps_rtmsupport('StopFcn',gcbh);  mask(Breaker){InitialState=InitialState, SwitchingTimes=[ 1/60  5/60 ], External=on, BreakerResistance=BreakerResistance, SnubberResistance=SnubberResistance, SnubberCapacitance=SnubberCapacitance, Measurements=None, MoreParameters=off, NoBreakLoop=off}
      mask prompts: InitialState "Initial status:"; SwitchingTimes "Switching times (s):"; BreakerResistance "Breaker resistance Ron (Ohm):"; SnubberResistance "Snubber resistance Rs (Ohm):"; SnubberCapacitance "Snubber capacitance Cs (F):"; MoreParameters "obsolete"; NoBreakLoop "Enable zero crossing detection (create an algebraic loop)"
      mask help: Implements a circuit breaker. When the external switching time option is selected, a Simulink logical signal is used to control the breaker operation.
      mask init: same as microgridLib/Fault /Fault A
      settings: CopyFcn=sps_rtmsupport('CopyFcn',gcbh); powericon('SwitchesCopyFcn','Breaker',gcb)  DeleteFcn=sps_rtmsupport('DeleteFcn',gcbh);  UndoDeleteFcn=sps_rtmsupport('UndoDeleteFcn',gcbh);  ModelCloseFcn=sps_rtmsupport('ModelCloseFcn',gcbh);  PreSaveFcn=sps_rtmsupport('PreSaveFcn',gcbh);  PostSaveFcn=sps_rtmsupport('PostSaveFcn',gcbh);  NameChangeFcn=sps_rtmsupport('NameChangeFcn',gcbh);  PreCopyFcn=sps_rtmsupport('PreCopyFcn',gcbh);  OpenFcn=sps_rtmsupport('OpenFcn',gcbh, [3 7 8 9]);  CloseFcn=sps_rtmsupport('CloseFcn',gcbh);  PreDeleteFcn=sps_rtmsupport('PreDeleteFcn',gcbh);
      mask Help: helpview(psbhelp);
      mask Callback External: powericon('BreakerCback',gcb);
      mask Callback BreakerResistance: powericon('SwitchesEnables',gcb,'Breaker');
      mask TypeOptions Measurements: None | Branch voltage | Branch current | Branch voltage and current
      mask Display: % plot(X.p1,Y.p1,X.p2,Y.p2,X.p3,Y.p3,X.p4,Y.p4,X.p5,Y.p5,X.p6,Y.p6)
  Breaker C : Subsystem  DialogController=POWERSYS.PowerSysDialog  LoadFcn=sps_rtmsupport('LoadFcn',gcbh);  StartFcn=sps_rtmsupport('StartFcn',gcbh);  StopFcn=sps_rtmsupport('StopFcn',gcbh);  mask(Breaker){InitialState=InitialState, SwitchingTimes=[ 1/60  5/60 ], External=on, BreakerResistance=BreakerResistance, SnubberResistance=SnubberResistance, SnubberCapacitance=SnubberCapacitance, Measurements=None, MoreParameters=off, NoBreakLoop=off}
      mask prompts: InitialState "Initial status:"; SwitchingTimes "Switching times (s):"; BreakerResistance "Breaker resistance Ron (Ohm):"; SnubberResistance "Snubber resistance Rs (Ohm):"; SnubberCapacitance "Snubber capacitance Cs (F):"; MoreParameters "obsolete"; NoBreakLoop "Enable zero crossing detection (create an algebraic loop)"
      mask help: Implements a circuit breaker. When the external switching time option is selected, a Simulink logical signal is used to control the breaker operation.
      mask init: same as microgridLib/Fault /Fault A
      settings: CopyFcn=sps_rtmsupport('CopyFcn',gcbh); powericon('SwitchesCopyFcn','Breaker',gcb)  DeleteFcn=sps_rtmsupport('DeleteFcn',gcbh);  UndoDeleteFcn=sps_rtmsupport('UndoDeleteFcn',gcbh);  ModelCloseFcn=sps_rtmsupport('ModelCloseFcn',gcbh);  PreSaveFcn=sps_rtmsupport('PreSaveFcn',gcbh);  PostSaveFcn=sps_rtmsupport('PostSaveFcn',gcbh);  NameChangeFcn=sps_rtmsupport('NameChangeFcn',gcbh);  PreCopyFcn=sps_rtmsupport('PreCopyFcn',gcbh);  OpenFcn=sps_rtmsupport('OpenFcn',gcbh, [3 7 8 9]);  CloseFcn=sps_rtmsupport('CloseFcn',gcbh);  PreDeleteFcn=sps_rtmsupport('PreDeleteFcn',gcbh);
      mask Help: helpview(psbhelp);
      mask Callback External: powericon('BreakerCback',gcb);
      mask Callback BreakerResistance: powericon('SwitchesEnables',gcb,'Breaker');
      mask TypeOptions Measurements: None | Branch voltage | Branch current | Branch voltage and current
      mask Display: % plot(X.p1,Y.p1,X.p2,Y.p2,X.p3,Y.p3,X.p4,Y.p4,X.p5,Y.p5,X.p6,Y.p6)
  C4 : Constant  Value=External
  Constant1 : Constant  Value=SwitchA
  Constant2 : Constant  Value=SwitchB
  Constant3 : Constant  Value=SwitchC
  Constant5 : Constant  Value=InitialState
  Stair Generator : spsStairGeneratorLib/Stair Generator  t=Switch_Times  e=SwitchStatus  Ts=Ts
  Switch : Switch  Threshold=0.5  ZeroCross=off  SaturateOnIntegerOverflow=off
  Switch1 : Switch  Threshold=0.5  ZeroCross=off  SaturateOnIntegerOverflow=off
  Switch2 : Switch  Threshold=0.5  ZeroCross=off  SaturateOnIntegerOverflow=off
  Switch3 : Switch  Threshold=0.5  ZeroCross=off  SaturateOnIntegerOverflow=off  InputSameDT=off
  ThreePhaseBreaker : PMComponent  PhysicalDomain=powersysdomain  LeftPortType=p1  RightPortType=p1  LConnTagsString=A|B|C  RConnTagsString=a|b|c  mask(InnerPowersysBlock){}
  A : PMIOPort  Side=Left
  B : PMIOPort  Port=2  Side=Left
  C : PMIOPort  Port=3  Side=Left
  a : PMIOPort  Port=4  Side=Right
  b : PMIOPort  Port=5  Side=Right
  c : PMIOPort  Port=6  Side=Right
  wires:
  Switch3/1 -> Switch2/1, Switch1/1, Switch/1
  Constant1/1 -> Switch/2
  Switch/1 -> Breaker A/1(c)
  Constant3/1 -> Switch2/2
  Switch2/1 -> Breaker C/1(c)
  Constant2/1 -> Switch1/2
  Switch1/1 -> Breaker B/1(c)
  C4/1 -> Switch3/2
  com/1 -> Switch3/1
  Stair Generator/1 -> Switch3/3
  Constant5/1 -> Switch/3, Switch1/3, Switch2/3
  connections:
  Breaker A/LConn1 -- ThreePhaseBreaker/RConn1 -- A/RConn1
  ThreePhaseBreaker/RConn2 -- Breaker B/LConn1 -- B/RConn1
  ThreePhaseBreaker/RConn3 -- Breaker C/LConn1 -- C/RConn1
  a/RConn1 -- ThreePhaseBreaker/LConn1 -- Breaker A/RConn1
  ThreePhaseBreaker/LConn2 -- Breaker B/RConn1 -- b/RConn1
  ThreePhaseBreaker/LConn3 -- Breaker C/RConn1 -- c/RConn1

== system microgridLib/Dynamic Load/Calculate Current/Break Algebraic Loop1 ==
  In1 : Inport
  1/Tr : Gain  Gain=1/Tau  SampleTime=Ts
  Discrete-Time Integrator : DiscreteIntegrator  SampleTime=Ts  ICPrevOutput=DiscIntNeverNeededParam  ICPrevScaledInput=DiscIntNeverNeededParam
  Sum : Sum  Inputs=|+-
  Out1 : Outport
  wires:
  Sum/1 -> 1/Tr/1
  1/Tr/1 -> Discrete-Time Integrator/1
  Discrete-Time Integrator/1 -> Sum/2, Out1/1
  In1/1 -> Sum/1

== system microgridLib/Dynamic Load/Calculate Current/Flag Current ==
  |V| : Inport
  Logical Operator : Logic  Operator=OR  AllPortsSameDT=off  OutDataTypeStr=boolean
  Max Voltage : Constant  Value=1.5*Vrms/sqrt(3)
  Min Voltage : Constant  Value=0.5*Vrms/sqrt(3)
  Relational Operator : RelationalOperator  Operator=>  OutDataTypeStr=boolean  RndMeth=Simplest  InputSameDT=off
  Relational Operator1 : RelationalOperator  Operator=<  OutDataTypeStr=boolean  RndMeth=Simplest  InputSameDT=off
  SinkOff : Outport
  wires:
  Max Voltage/1 -> Relational Operator/2
  Relational Operator1/1 -> Logical Operator/2
  Min Voltage/1 -> Relational Operator1/2
  Relational Operator/1 -> Logical Operator/1
  Logical Operator/1 -> SinkOff/1
  |V|/1 -> Relational Operator/1, Relational Operator1/1

== system microgridLib/Dynamic Load (Modified SPS)/Three-Phase Dynamic Load/Measurement list ==
  In1 : Inport
  Bus Creator1 : BusCreator  Inputs=3
  Demux : Demux  Outputs=[1,1,1]
  Out1 : Outport
  wires:
  Demux/3 -> Bus Creator1/3  "Reactive power Q (var)"
  Demux/1 -> Bus Creator1/1  "Positive-sequence voltage V (pu)"
  Demux/2 -> Bus Creator1/2  "Active power P (W)"
  Bus Creator1/1 -> Out1/1
  In1/1 -> Demux/1

== system microgridLib/Dynamic Load (Modified SPS)/Three-Phase Dynamic Load (custom)/Measurement list ==
  In1 : Inport
  Bus Creator1 : BusCreator  Inputs=3
  Demux : Demux  Outputs=[1,1,1]
  Out1 : Outport
  wires:
  In1/1 -> Demux/1
  Bus Creator1/1 -> Out1/1
  Demux/2 -> Bus Creator1/2  "Active power P (W)"
  Demux/1 -> Bus Creator1/1  "Positive-sequence voltage V (pu)"
  Demux/3 -> Bus Creator1/3  "Reactive power Q (var)"

== system microgridLib/Dynamic Load (Modified SPS)/Three-Phase Dynamic Load (custom)/Model ==
  v : Inport  PortDimensions=2
  PQ : Inport  Port=2  PortDimensions=2
  Complex to Real-Imag : ComplexToRealImag
  Demux : Demux  Outputs=2
      settings: DisplayOption=none
  Discrete 3-phase PLL : Subsystem  mask(Discrete 3-phase PLL){Par_Init=[Pha_V0  fnom], ParK=[60 1400], Ts=Ts}
      mask prompts: Par_Init "Initial inputs:[ Phase(degrees)   Frequency(Hz) ]"; ParK "Regulator gains [ Kp  Ki ]"; Ts "Sample time:"
      mask init:
      | Kp=ParK(1);
      | Ki=ParK(2);
      | Phase_Init=Par_Init(1);
      | Finit=Par_Init(2);
  Ground : Ground
  Mean (Variable Frequency) : spsMeanVariableFrequencyLib/Mean (Variable Frequency)  Finit=fnom  Fmin=45  Vinit=Mag_V0  Ts=Ts
      settings: LibrarySourceBlock=|
      | sps_lib/Sensors and Measurements/Mean
      | (Variable Frequency)
  Mean (Variable Frequency)1 : spsMeanVariableFrequencyLib/Mean (Variable Frequency)  Finit=fnom  Fmin=45  Vinit=0  Ts=Ts
      settings: LibrarySourceBlock=|
      | sps_lib/Sensors and Measurements/Mean
      | (Variable Frequency)
  Mux1 : Mux  Inputs=3
  Positive Sequence current : Subsystem
  Real-Imag to Complex : RealImagToComplex
  Real-Imag to Complex1 : RealImagToComplex
  Selector : Selector  InputPortWidth=3  IndexOptions=Index vector (dialog)  Indices=1:2  OutputSizes=1
  Unit Delay1 : UnitDelay  InitialCondition=I1_init*exp(-j*Pha_V0*pi/180)  SampleTime=Ts  HasFrameUpgradeWarning=on
  V> pu : Gain  Gain=1/Vbase  SaturateOnIntegerOverflow=on  OutDataTypeStr=Inherit: Same as input  ParamDataTypeStr=Inherit: Same as input
  dq0 to abc : spsdq0toabcLib/dq0 to abc  Alignment=90 degrees behind phase A axis
  i : Outport
  m : Outport  Port=2
  wires:
  dq0 to abc/1 -> Selector/1
  Selector/1 -> i/1
  v/1 -> V> pu/1
  V> pu/1 -> Discrete 3-phase PLL/1(Vab_bc (pu))
  Real-Imag to Complex/1 -> Positive Sequence current/1(V1(pu))
  Mux1/1 -> dq0 to abc/1
  Positive Sequence current/1(I1(A)) -> Unit Delay1/1
  Discrete 3-phase PLL/3(Vq) -> Mean (Variable Frequency)1/2
  Ground/1 -> Mux1/3
  Mean (Variable Frequency)/1 -> Real-Imag to Complex/1
  Mean (Variable Frequency)1/1 -> Real-Imag to Complex/2
  Complex to Real-Imag/1 -> Mux1/1
  Complex to Real-Imag/2 -> Mux1/2
  Discrete 3-phase PLL/2(Vd) -> Mean (Variable Frequency)/2
  Discrete 3-phase PLL/4(wt) -> dq0 to abc/2
  Discrete 3-phase PLL/1(Freq) -> Mean (Variable Frequency)/1, Mean (Variable Frequency)1/1
  PQ/1 -> Demux/1
  Demux/1 -> Real-Imag to Complex1/1
  Demux/2 -> Real-Imag to Complex1/2
  Real-Imag to Complex1/1 -> Positive Sequence current/2(S_ext)
  Positive Sequence current/2(VPQ) -> m/1
  Unit Delay1/1 -> Complex to Real-Imag/1

== system microgridLib/Dynamic Load1/Calculate Current/Break Algebraic Loop1 ==
  In1 : Inport
  1/Tr : Gain  Gain=1/Tau  SampleTime=Ts
  Discrete-Time Integrator : DiscreteIntegrator  SampleTime=Ts  ICPrevOutput=DiscIntNeverNeededParam  ICPrevScaledInput=DiscIntNeverNeededParam
  Sum : Sum  Inputs=|+-
  Out1 : Outport
  wires:
  In1/1 -> Sum/1
  Discrete-Time Integrator/1 -> Out1/1, Sum/2
  1/Tr/1 -> Discrete-Time Integrator/1
  Sum/1 -> 1/Tr/1

== system microgridLib/Dynamic Load1/Calculate Current/Flag Current ==
  |V| : Inport
  Logical Operator : Logic  Operator=OR  AllPortsSameDT=off  OutDataTypeStr=boolean
  Max Voltage : Constant  Value=1.5*Vrms/sqrt(3)
  Min Voltage : Constant  Value=0.5*Vrms/sqrt(3)
  Relational Operator : RelationalOperator  Operator=>  OutDataTypeStr=boolean  RndMeth=Simplest  InputSameDT=off
  Relational Operator1 : RelationalOperator  Operator=<  OutDataTypeStr=boolean  RndMeth=Simplest  InputSameDT=off
  SinkOff : Outport
  wires:
  |V|/1 -> Relational Operator1/1, Relational Operator/1
  Logical Operator/1 -> SinkOff/1
  Relational Operator/1 -> Logical Operator/1
  Min Voltage/1 -> Relational Operator1/2
  Relational Operator1/1 -> Logical Operator/2
  Max Voltage/1 -> Relational Operator/2

== system microgridLib/Fault /Fault A/Model ==
  "gate " : Inport
  Uswitch : Inport  Port=2
  C4 : Constant  Value=BR.com
  Data Type Conversion : DataTypeConversion  OutDataTypeStr=double
  Switch3 : Switch  Threshold=0.5  ZeroCross=off  SaturateOnIntegerOverflow=off
  This signal is not used : Terminator
  Timer : Subsystem  DialogController=POWERSYS.PowerSysDialog  mask(Timer){t=BR.SwitchingTimes, e=BR.switchings}
      mask prompts: t "Time (s):"; e "Amplitude:"
      mask help:
      | Generates a signal changing at specified times.
      |
      | If a signal value is not specified at time zero, the output is kept at 0 until the first specified transition time.
      mask init:
      | tt=t;
      | sv=e;
      | if isempty(tt) | isempty(sv)
      | 	% probably during the load process when under a masked block.
      | 	tt=0;
      | 	sv=1;
      | end
      | %
      | if length(sv) ~= length(tt),
      |    Erreur.message = 'The vectors specifying the time and amplitude pairs must have the same length.';
      |    Erreur.identifier = 'SimscapePowerSystemsST:TimerBlock:ParameterError';
      |    powericon('psberror',Erreur.message,Erreur.identifier,'NoUiwait');
      | end
      | if tt(1)~=0,
      |    tt=[0 tt];
      |    sv=[~sv(1) sv];
      | end
      | n=length(tt);
      | vec_dt=[tt,0]-[0,tt] ;
      | vec_dt=vec_dt(2:n);
      | if any(vec_dt<=0)
      |    Erreur.message = 'All transition times must be in increasing order.';
      |    Erreur.identifier = 'SimscapePowerSystemsST:TimerBlock:ParameterError';
      |    powericon('psberror',Erreur.message,Erreur.identifier,'NoUiwait');
      | end
      | tv=[-1,tt(1),reshape(repmat(reshape(tt(2:end),1,length(tt)-1),2,1),1,2*length(tt)-2),tt(end)+1];
      | %sv=(sv(:)'~=0);
      | opv=[sv(1),reshape(repmat(sv(1:end-1),2,1),1,2*length(sv)-2),sv(end),sv(end)];
      | 
      | power_initmask();
      mask Help: helpview(psbhelp)
      mask Display: plot( tv(2:end-1), opv(2:end-1) )
  gate : Outport
  wires:
  "gate "/1 -> Data Type Conversion/1
  Switch3/1 -> gate/1
  Data Type Conversion/1 -> Switch3/1
  Timer/1(Out) -> Switch3/3
  C4/1 -> Switch3/2
  Uswitch/1 -> This signal is not used/1

== system microgridLib/Fault /Fault B/Model ==
  "gate " : Inport
  Uswitch : Inport  Port=2
  C4 : Constant  Value=BR.com
  Data Type Conversion : DataTypeConversion  OutDataTypeStr=double
  Switch3 : Switch  Threshold=0.5  ZeroCross=off  SaturateOnIntegerOverflow=off
  This signal is not used : Terminator
  Timer : Subsystem  DialogController=POWERSYS.PowerSysDialog  mask(Timer){t=BR.SwitchingTimes, e=BR.switchings}
      mask prompts: t "Time (s):"; e "Amplitude:"
      mask help:
      | Generates a signal changing at specified times.
      |
      | If a signal value is not specified at time zero, the output is kept at 0 until the first specified transition time.
      mask init: same as microgridLib/Fault /Fault A/Model/Timer
      mask Help: helpview(psbhelp)
      mask Display: plot( tv(2:end-1), opv(2:end-1) )
  gate : Outport
  wires:
  "gate "/1 -> Data Type Conversion/1
  Switch3/1 -> gate/1
  Data Type Conversion/1 -> Switch3/1
  Timer/1(Out) -> Switch3/3
  C4/1 -> Switch3/2
  Uswitch/1 -> This signal is not used/1
